simulink model "WiperSystem"  (R2022b)
settings: Solver=ode4  StartTime=0.0  StopTime=20  RelTol=1e-3
undefined symbols (not defined in the file): sigbuilder_block
libraries: eeGeneralControl x1, simulink x1
settings Model: Creator=AymanLaptop  LastModifiedBy=AymanLaptop
settings OptimizationCC: DefaultParameterBehavior=Inlined  GainParamInheritBuiltInType=on  UseFloatMulNetSlope=on  InlineInvariantSignals=on  EfficientFloat2IntCast=on
settings RTWCC: BuildConfiguration=Faster Runs
settings GRTTargetCC: MatFileLogging=off  SupportNonFinite=off

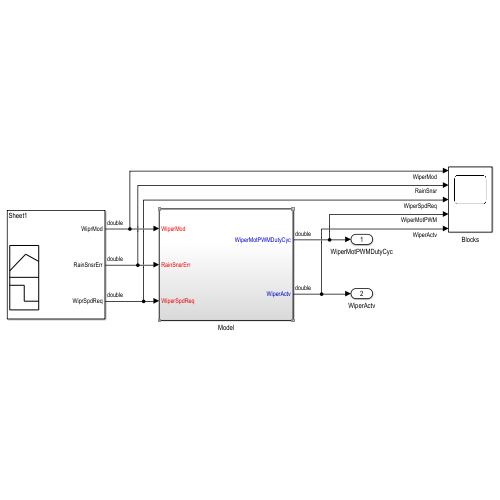
[thumbnail: Simulink's stored preview of the top-level diagram]
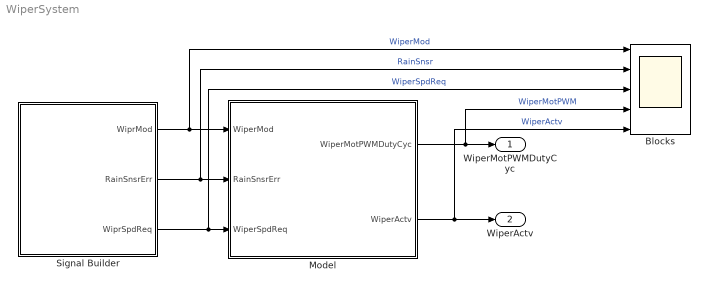
== system WiperSystem ==
  Blocks : Scope  NumInputPorts=5
  Model : Subsystem
  Signal Builder : Subsystem  Tag=STV Subsys  LoadFcn=sigbuilder_block('load');  StartFcn=sigbuilder_block('start');  StopFcn=sigbuilder_block('stop');  ClipboardFcn=sigbuilder_block('clipboard');  mask(Sigbuilder block){tuvar=[0:10]}
      mask help: Simulink:masks:SigbuilderBlock_MD
      mask init:
      | if ~strcmp(get_param(bdroot(gcbh),'SimulationStatus'),'stopped') tuvar = sigbuilder_block('maskInit'); end
      settings: CopyFcn=sigbuilder_block('copy');  DeleteFcn=sigbuilder_block('delete');  ModelCloseFcn=sigbuilder_block('modelClose');  PreSaveFcn=sigbuilder_block('preSave');  PauseFcn=sigbuilder_block('pause');  ContinueFcn=sigbuilder_block('continue');  NameChangeFcn=sigbuilder_block('namechange');  OpenFcn=sigbuilder_block('open',[6 0 1012.5 455.25 ]);  CloseFcn=sigbuilder_block('close');
      mask Display: plot(0, 0, 100, 100,[2, 2, 32, 32, 2], [68, 8, 8, 68, 68],[32, 2], [38, 38], [32, 19, 2],[53, 60, 44], [32, 17, 17, 2],[16, 16, 31, 31]);txt = getActiveGroup(gcbh);text(2, 100, txt,'verticalAlignment', 'top');
  WiperMotPWMDutyCyc : Outport
  WiperActv : Outport  Port=2
  wires:
  Model/1(WiperMotPWMDutyCyc) -> Blocks/4, WiperMotPWMDutyCyc/1  "WiperMotPWM"
  Model/2(WiperActv) -> Blocks/5, WiperActv/1  "WiperActv"
  Signal Builder/1(WiprMod) -> Model/1(WiperMod), Blocks/1  "WiperMod"
  Signal Builder/2(RainSnsrErr) -> Blocks/2, Model/2(RainSnsrErr)  "RainSnsr"
  Signal Builder/3(WiprSpdReq) -> Blocks/3, Model/3(WiperSpdReq)  "WiperSpdReq"

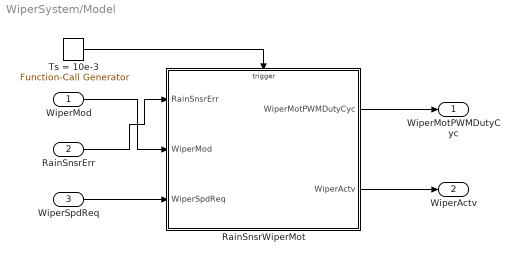
== system WiperSystem/Model ==
  WiperMod : Inport
  RainSnsrErr : Inport  Port=2
  WiperSpdReq : Inport  Port=3
  RainSnsrWiperMot : Subsystem
  Ts = 10e-3 : simulink/Ports & Subsystems/Function-Call Generator  sample_time=10e-3  numberOfIterations=1  DisallowWideOutput=off
  WiperMotPWMDutyCyc : Outport
  WiperActv : Outport  Port=2
  wires:
  Ts = 10e-3/1 -> RainSnsrWiperMot/Trigger
  RainSnsrWiperMot/2(WiperActv) -> WiperActv/1
  RainSnsrErr/1 -> RainSnsrWiperMot/1(RainSnsrErr)
  RainSnsrWiperMot/1(WiperMotPWMDutyCyc) -> WiperMotPWMDutyCyc/1
  WiperSpdReq/1 -> RainSnsrWiperMot/3(WiperSpdReq)
  WiperMod/1 -> RainSnsrWiperMot/2(WiperMod)

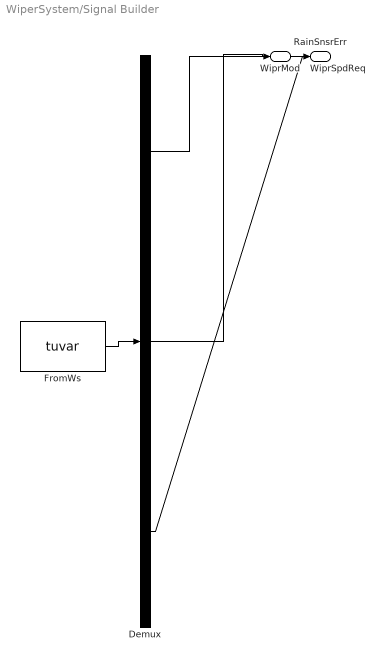
== system WiperSystem/Signal Builder ==
  Demux : Demux  Tag=STV Demux  Outputs=3
      settings: DisplayOption=none
  FromWs : FromWorkspace  Tag=STV FromWs  VariableName=tuvar  SampleTime=1  OutputAfterFinalValue=Holding final value
      SigBuilderData=|
      | common.afterFinalStr = 'Hold final value'
      | common.sampleTime = '1'
      | dataSet.timeRange = [0 16]
      | dataSet.name = 'Sheet1'
      | sbobj.Groups.Name = 'Sheet1'
      | sbobj.Groups.Signals(1).Name = 'WiprMod'
      | sbobj.Groups.Signals(1).XData = [0 1 2 3 4 5 6 7 8 9 10 11 12 13 14 15 16]
      | sbobj.Groups.Signals(1).YData = [0 0 2 2 3 3 1 1 1 1 1 1 1 1 1 1 1]
      | sbobj.Groups.Signals(2).Name = 'RainSnsrErr'
      | sbobj.Groups.Signals(2).XData = [0 1 2 3 4 5 6 7 8 9 10 11 12 13 14 15 16]
      | sbobj.Groups.Signals(2).YData = [0 0 0 0 0 0 0 0 0 0 0 0 0 0 0 1 0]
      | sbobj.Groups.Signals(3).Name = 'WiprSpdReq'
      | sbobj.Groups.Signals(3).XData = [0 1 2 3 4 5 6 7 8 9 10 11 12 13 14 15 16]
      | sbobj.Groups.Signals(3).YData = [0 0 0 0 0 0 0 0 1 2 3 4 5 6 7 7 7]
      | sbobj.Groups.TimeRange = [0 16]
  WiprMod : Outport  Tag=STV Outport
  RainSnsrErr : Outport  Tag=STV Outport  Port=2
  WiprSpdReq : Outport  Tag=STV Outport  Port=3
  wires:
  Demux/1 -> WiprMod/1
  FromWs/1 -> Demux/1
  Demux/2 -> RainSnsrErr/1
  Demux/3 -> WiprSpdReq/1

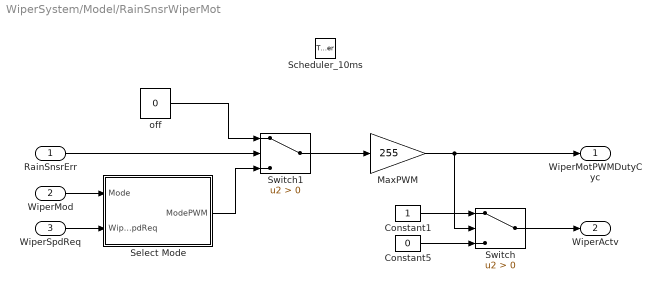
== system WiperSystem/Model/RainSnsrWiperMot ==
  RainSnsrErr : Inport
  WiperMod : Inport  Port=2
  WiperSpdReq : Inport  Port=3
  Scheduler_10ms : TriggerPort  TriggerType=function-call  VariantControl=(inherit)
  Constant1 : Constant
  Constant5 : Constant  Value=0
  MaxPWM : Gain  Gain=255
  Select Mode : Subsystem
  Switch : Switch  Criteria=u2 > Threshold  SaturateOnIntegerOverflow=off  InputSameDT=off
  Switch1 : Switch  Criteria=u2 > Threshold  SaturateOnIntegerOverflow=off  InputSameDT=off
  off : Constant  Value=0
  WiperMotPWMDutyCyc : Outport
  WiperActv : Outport  Port=2
  wires:
  MaxPWM/1 -> WiperMotPWMDutyCyc/1, Switch/2
  Constant1/1 -> Switch/1
  Constant5/1 -> Switch/3
  Switch/1 -> WiperActv/1
  RainSnsrErr/1 -> Switch1/2
  Select Mode/1(ModePWM) -> Switch1/3
  Switch1/1 -> MaxPWM/1
  off/1 -> Switch1/1
  WiperMod/1 -> Select Mode/1(Mode)
  WiperSpdReq/1 -> Select Mode/2(WiperSpdReq)

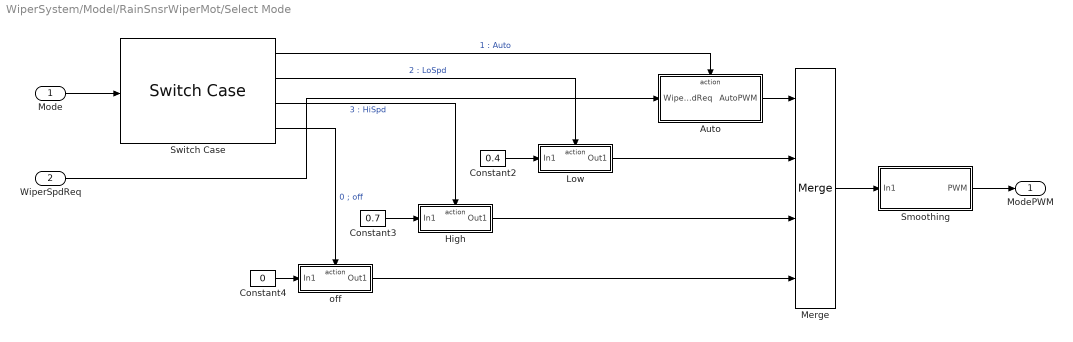
== system WiperSystem/Model/RainSnsrWiperMot/Select Mode ==
  Mode : Inport
  WiperSpdReq : Inport  Port=2
  Auto : Subsystem  TreatAsAtomicUnit=on
  Constant2 : Constant  Value=0.4
  Constant3 : Constant  Value=0.7
  Constant4 : Constant  Value=0
  High : Subsystem  TreatAsAtomicUnit=on
  Low : Subsystem  TreatAsAtomicUnit=on
  Merge : Merge  Inputs=4
  Smoothing : Subsystem
  Switch Case : SwitchCase  CaseConditions={1, 2, 3}
  off : Subsystem  TreatAsAtomicUnit=on
  ModePWM : Outport
  wires:
  Switch Case/1 -> Auto/Action  "1 : Auto"
  WiperSpdReq/1 -> Auto/1(WiperSpdReq)
  Constant3/1 -> High/1(In1)
  Auto/1(AutoPWM) -> Merge/1
  Switch Case/2 -> Low/Action  "2 : LoSpd"
  Switch Case/3 -> High/Action  "3 : HiSpd"
  Constant2/1 -> Low/1(In1)
  Switch Case/4 -> off/Action  "0 ; off"
  Constant4/1 -> off/1(In1)
  High/1(Out1) -> Merge/3
  off/1(Out1) -> Merge/4
  Low/1(Out1) -> Merge/2
  Merge/1 -> Smoothing/1(In1)
  Mode/1 -> Switch Case/1
  Smoothing/1(PWM) -> ModePWM/1

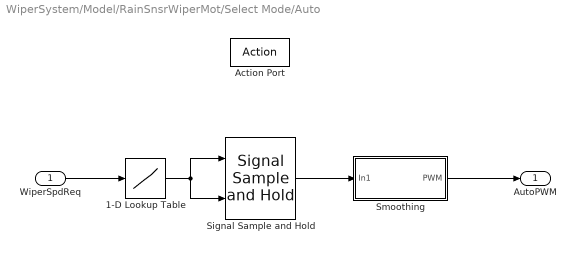
== system WiperSystem/Model/RainSnsrWiperMot/Select Mode/Auto ==
  WiperSpdReq : Inport
  Action Port : ActionPort  ActionPortLabel=case [ 1 ]:
  1-D Lookup Table : Lookup_n-D  NumberOfTableDimensions=1  BreakpointsForDimension1=[0 1 2 3 4 5 6 7]  Table=[0 0.40 0.45 0.50 0.55 0.60 0.65 0.70]  DiagnosticForOutOfRangeInput=Warning  RemoveProtectionInput=on  InternalRulePriority=Speed  RndMeth=Simplest
  Signal Sample and Hold : eeGeneralControl/Signal Sample and Hold  LabelModeActiveChoice=Discrete  x0=0  Ts=-1
      settings: LibrarySourceBlock=ee_sl_lib/General Control/Signal Sample and Hold
  Smoothing : Subsystem
  AutoPWM : Outport
  wires:
  Smoothing/1(PWM) -> AutoPWM/1
  1-D Lookup Table/1 -> Signal Sample and Hold/1, Signal Sample and Hold/2
  WiperSpdReq/1 -> 1-D Lookup Table/1
  Signal Sample and Hold/1 -> Smoothing/1(In1)

== system WiperSystem/Model/RainSnsrWiperMot/Select Mode/High ==
  In1 : Inport
  Action Port : ActionPort  ActionPortLabel=case [ 3 ]:
  Out1 : Outport
  wires:
  In1/1 -> Out1/1

== system WiperSystem/Model/RainSnsrWiperMot/Select Mode/Low ==
  In1 : Inport
  Action Port : ActionPort  ActionPortLabel=case [ 2 ]:
  Out1 : Outport
  wires:
  In1/1 -> Out1/1

== system WiperSystem/Model/RainSnsrWiperMot/Select Mode/Smoothing ==
  In1 : Inport
  Change Speed : Subsystem
  Resettable Delay : Delay  DelayLength=1  InitialConditionSource=Input port
      settings: InputPortMap=u0,p4
  PWM : Outport
  wires:
  Change Speed/1(PWM) -> PWM/1, Resettable Delay/1
  In1/1 -> Resettable Delay/2, Change Speed/1(req)
  Resettable Delay/1 -> Change Speed/2(prev)  "prev"

== system WiperSystem/Model/RainSnsrWiperMot/Select Mode/off ==
  In1 : Inport
  Action Port : ActionPort  ActionPortLabel=default:
  Out1 : Outport
  wires:
  In1/1 -> Out1/1

== system WiperSystem/Model/RainSnsrWiperMot/Select Mode/Auto/Smoothing ==
  In1 : Inport
  Change Speed : Subsystem
  Resettable Delay : Delay  DelayLength=1  InitialConditionSource=Input port
      settings: InputPortMap=u0,p4
  PWM : Outport
  wires:
  Change Speed/1(PWM) -> PWM/1, Resettable Delay/1
  In1/1 -> Resettable Delay/2, Change Speed/1(req)
  Resettable Delay/1 -> Change Speed/2(prev)  "prev"

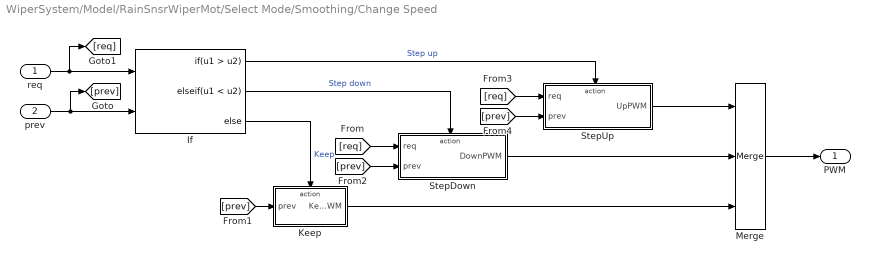
== system WiperSystem/Model/RainSnsrWiperMot/Select Mode/Smoothing/Change Speed ==
  req : Inport
  prev : Inport  Port=2
  If : If  NumInputs=2  IfExpression=u1 > u2  ElseIfExpressions=u1 < u2
  Keep : Subsystem  TreatAsAtomicUnit=on
  Merge : Merge  Inputs=3
  StepDown : Subsystem  TreatAsAtomicUnit=on
  StepUp : Subsystem  TreatAsAtomicUnit=on
  PWM : Outport
  wires:
  [req] -> StepUp/1(req)
  If/2 -> StepDown/Action  "Step down"
  StepDown/1(DownPWM) -> Merge/2
  [prev] -> Keep/1(prev)
  [prev] -> StepDown/2(prev)
  If/3 -> Keep/Action  "Keep"
  prev/1 -> [prev], If/2
  req/1 -> [req], If/1
  StepUp/1(UpPWM) -> Merge/1
  If/1 -> StepUp/Action  "Step up"
  [req] -> StepDown/1(req)
  [prev] -> StepUp/2(prev)
  Merge/1 -> PWM/1
  Keep/1(KeepPWM) -> Merge/3

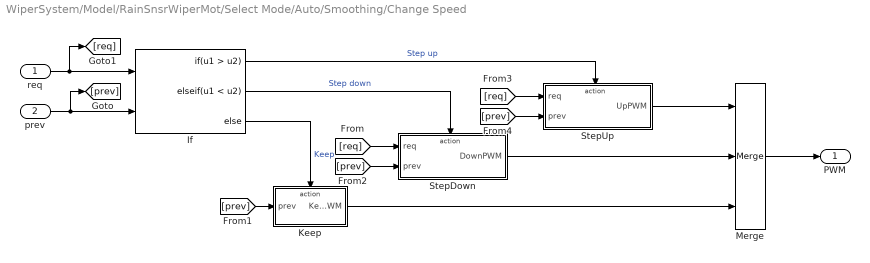
== system WiperSystem/Model/RainSnsrWiperMot/Select Mode/Auto/Smoothing/Change Speed ==
  req : Inport
  prev : Inport  Port=2
  If : If  NumInputs=2  IfExpression=u1 > u2  ElseIfExpressions=u1 < u2
  Keep : Subsystem  TreatAsAtomicUnit=on
  Merge : Merge  Inputs=3
  StepDown : Subsystem  TreatAsAtomicUnit=on
  StepUp : Subsystem  TreatAsAtomicUnit=on
  PWM : Outport
  wires:
  [req] -> StepUp/1(req)
  If/2 -> StepDown/Action  "Step down"
  StepDown/1(DownPWM) -> Merge/2
  [prev] -> Keep/1(prev)
  [prev] -> StepDown/2(prev)
  If/3 -> Keep/Action  "Keep"
  prev/1 -> [prev], If/2
  req/1 -> [req], If/1
  StepUp/1(UpPWM) -> Merge/1
  If/1 -> StepUp/Action  "Step up"
  [req] -> StepDown/1(req)
  [prev] -> StepUp/2(prev)
  Merge/1 -> PWM/1
  Keep/1(KeepPWM) -> Merge/3

== system WiperSystem/Model/RainSnsrWiperMot/Select Mode/Smoothing/Change Speed/Keep ==
  prev : Inport
  Action Port : ActionPort  ActionPortLabel=else
  KeepPWM : Outport
  wires:
  prev/1 -> KeepPWM/1

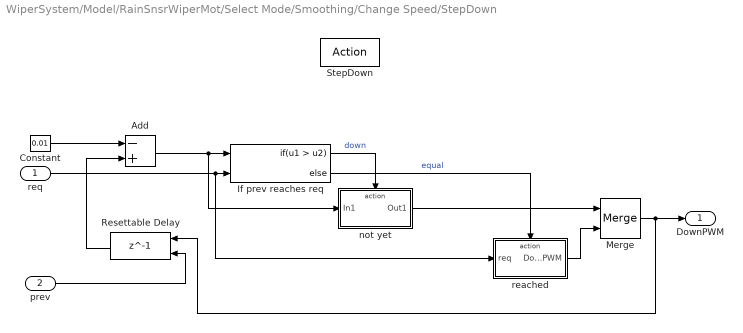
== system WiperSystem/Model/RainSnsrWiperMot/Select Mode/Smoothing/Change Speed/StepDown ==
  req : Inport
  prev : Inport  Port=2
  StepDown : ActionPort  ActionPortLabel=elseif(u1 < u2)
  Add : Sum  Inputs=-+
  Constant : Constant  Value=0.01
  If prev reaches req : If  NumInputs=2  IfExpression=u1 > u2
  Merge : Merge
  Resettable Delay : Delay  DelayLength=1  InitialConditionSource=Input port
      settings: InputPortMap=u0,p4
  not yet : Subsystem  TreatAsAtomicUnit=on
  reached : Subsystem  TreatAsAtomicUnit=on
  DownPWM : Outport
  wires:
  prev/1 -> Resettable Delay/2
  Constant/1 -> Add/1
  Resettable Delay/1 -> Add/2
  Add/1 -> not yet/1(In1), If prev reaches req/1
  req/1 -> reached/1(req), If prev reaches req/2
  If prev reaches req/1 -> not yet/Action  "down"
  not yet/1(Out1) -> Merge/1
  If prev reaches req/2 -> reached/Action  "equal"
  Merge/1 -> Resettable Delay/1, DownPWM/1
  reached/1(DownPWM) -> Merge/2

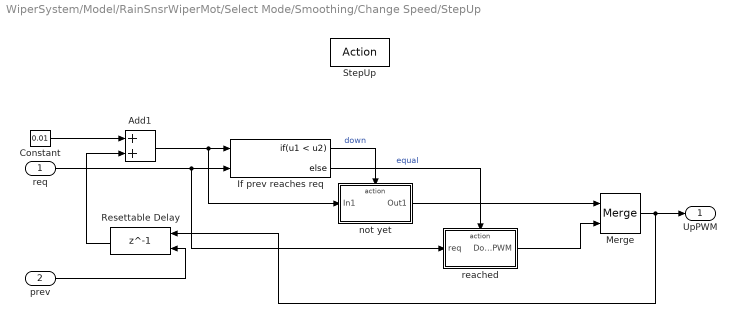
== system WiperSystem/Model/RainSnsrWiperMot/Select Mode/Smoothing/Change Speed/StepUp ==
  req : Inport
  prev : Inport  Port=2
  StepUp : ActionPort  ActionPortLabel=if(u1 > u2)
  Add1 : Sum
  Constant : Constant  Value=0.01
  If prev reaches req : If  NumInputs=2  IfExpression=u1 < u2
  Merge : Merge
  Resettable Delay : Delay  DelayLength=1  InitialConditionSource=Input port
      settings: InputPortMap=u0,p4
  not yet : Subsystem  TreatAsAtomicUnit=on
  reached : Subsystem  TreatAsAtomicUnit=on
  UpPWM : Outport
  wires:
  Add1/1 -> not yet/1(In1), If prev reaches req/1
  If prev reaches req/2 -> reached/Action  "equal"
  If prev reaches req/1 -> not yet/Action  "down"
  not yet/1(Out1) -> Merge/1
  Constant/1 -> Add1/1
  Resettable Delay/1 -> Add1/2
  req/1 -> reached/1(req), If prev reaches req/2
  prev/1 -> Resettable Delay/2
  reached/1(DownPWM) -> Merge/2
  Merge/1 -> UpPWM/1, Resettable Delay/1

== system WiperSystem/Model/RainSnsrWiperMot/Select Mode/Auto/Smoothing/Change Speed/Keep ==
  prev : Inport
  Action Port : ActionPort  ActionPortLabel=else
  KeepPWM : Outport
  wires:
  prev/1 -> KeepPWM/1

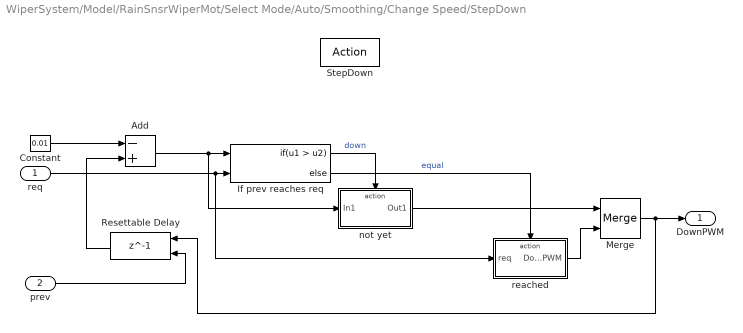
== system WiperSystem/Model/RainSnsrWiperMot/Select Mode/Auto/Smoothing/Change Speed/StepDown ==
  req : Inport
  prev : Inport  Port=2
  StepDown : ActionPort  ActionPortLabel=elseif(u1 < u2)
  Add : Sum  Inputs=-+
  Constant : Constant  Value=0.01
  If prev reaches req : If  NumInputs=2  IfExpression=u1 > u2
  Merge : Merge
  Resettable Delay : Delay  DelayLength=1  InitialConditionSource=Input port
      settings: InputPortMap=u0,p4
  not yet : Subsystem  TreatAsAtomicUnit=on
  reached : Subsystem  TreatAsAtomicUnit=on
  DownPWM : Outport
  wires:
  prev/1 -> Resettable Delay/2
  Constant/1 -> Add/1
  Resettable Delay/1 -> Add/2
  Add/1 -> not yet/1(In1), If prev reaches req/1
  req/1 -> reached/1(req), If prev reaches req/2
  If prev reaches req/1 -> not yet/Action  "down"
  not yet/1(Out1) -> Merge/1
  If prev reaches req/2 -> reached/Action  "equal"
  Merge/1 -> Resettable Delay/1, DownPWM/1
  reached/1(DownPWM) -> Merge/2

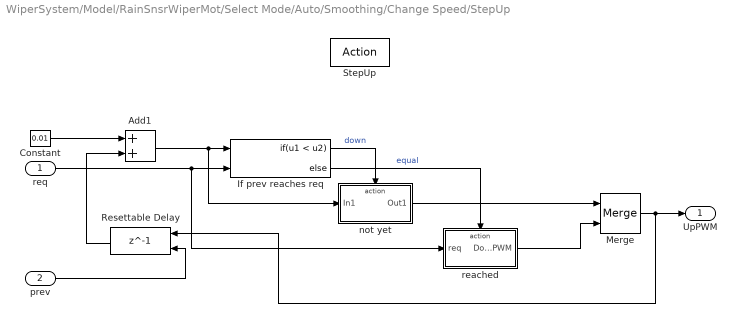
== system WiperSystem/Model/RainSnsrWiperMot/Select Mode/Auto/Smoothing/Change Speed/StepUp ==
  req : Inport
  prev : Inport  Port=2
  StepUp : ActionPort  ActionPortLabel=if(u1 > u2)
  Add1 : Sum
  Constant : Constant  Value=0.01
  If prev reaches req : If  NumInputs=2  IfExpression=u1 < u2
  Merge : Merge
  Resettable Delay : Delay  DelayLength=1  InitialConditionSource=Input port
      settings: InputPortMap=u0,p4
  not yet : Subsystem  TreatAsAtomicUnit=on
  reached : Subsystem  TreatAsAtomicUnit=on
  UpPWM : Outport
  wires:
  Add1/1 -> not yet/1(In1), If prev reaches req/1
  If prev reaches req/2 -> reached/Action  "equal"
  If prev reaches req/1 -> not yet/Action  "down"
  not yet/1(Out1) -> Merge/1
  Constant/1 -> Add1/1
  Resettable Delay/1 -> Add1/2
  req/1 -> reached/1(req), If prev reaches req/2
  prev/1 -> Resettable Delay/2
  reached/1(DownPWM) -> Merge/2
  Merge/1 -> UpPWM/1, Resettable Delay/1

== system WiperSystem/Model/RainSnsrWiperMot/Select Mode/Smoothing/Change Speed/StepDown/not yet ==
  In1 : Inport
  Action Port : ActionPort  ActionPortLabel=if(u1 > u2)
  Out1 : Outport
  wires:
  In1/1 -> Out1/1

== system WiperSystem/Model/RainSnsrWiperMot/Select Mode/Smoothing/Change Speed/StepDown/reached ==
  req : Inport
  Action Port : ActionPort  ActionPortLabel=else
  DownPWM : Outport
  wires:
  req/1 -> DownPWM/1

== system WiperSystem/Model/RainSnsrWiperMot/Select Mode/Smoothing/Change Speed/StepUp/not yet ==
  In1 : Inport
  Action Port : ActionPort  ActionPortLabel=if(u1 < u2)
  Out1 : Outport
  wires:
  In1/1 -> Out1/1

== system WiperSystem/Model/RainSnsrWiperMot/Select Mode/Smoothing/Change Speed/StepUp/reached ==
  req : Inport
  Action Port : ActionPort  ActionPortLabel=else
  DownPWM : Outport
  wires:
  req/1 -> DownPWM/1

== system WiperSystem/Model/RainSnsrWiperMot/Select Mode/Auto/Smoothing/Change Speed/StepDown/not yet ==
  In1 : Inport
  Action Port : ActionPort  ActionPortLabel=if(u1 > u2)
  Out1 : Outport
  wires:
  In1/1 -> Out1/1

== system WiperSystem/Model/RainSnsrWiperMot/Select Mode/Auto/Smoothing/Change Speed/StepDown/reached ==
  req : Inport
  Action Port : ActionPort  ActionPortLabel=else
  DownPWM : Outport
  wires:
  req/1 -> DownPWM/1

== system WiperSystem/Model/RainSnsrWiperMot/Select Mode/Auto/Smoothing/Change Speed/StepUp/not yet ==
  In1 : Inport
  Action Port : ActionPort  ActionPortLabel=if(u1 < u2)
  Out1 : Outport
  wires:
  In1/1 -> Out1/1

== system WiperSystem/Model/RainSnsrWiperMot/Select Mode/Auto/Smoothing/Change Speed/StepUp/reached ==
  req : Inport
  Action Port : ActionPort  ActionPortLabel=else
  DownPWM : Outport
  wires:
  req/1 -> DownPWM/1
